simulink model "delta_dynamics"  (R2018a)
settings: Solver=VariableStepAuto  StartTime=0.0  StopTime=10.0  RelTol=1e-3
values from neighbouring files (symbols this model uses):
  Ig = [1 0 0; 0 1 0; 0 0 1]    [HapticsSetup.m]    (also in delta_massMatrix.m = u(1:3,:); delta_nonlinearTerm.m = u(1:3,:))
  M = m*eye(3)*Im    [HapticsSetup.m]    (also in Mmatrix.m = (J')^(-1)*Aq*(J^-1); delta_nonlinearTerm.m = u(4:6,:))
  q0 = [0;0;0]    [HapticsSetup.m]
  x0 = interx(p(:,1),p(:,2),p(:,3),Lb,Lb,Lb,0)    [HapticsSetup.m]
  xd0 = [0;0;0]    [HapticsSetup.m]
undefined symbols (not defined in the file or in its folder): delta_massMatrix, delta_nonlinearTerm, deltaJacobian, derivative_deltaInvJacobian
settings Model: Creator=klay  LastModifiedBy=augus
settings CodeAppCC: StateflowObjectComments=on

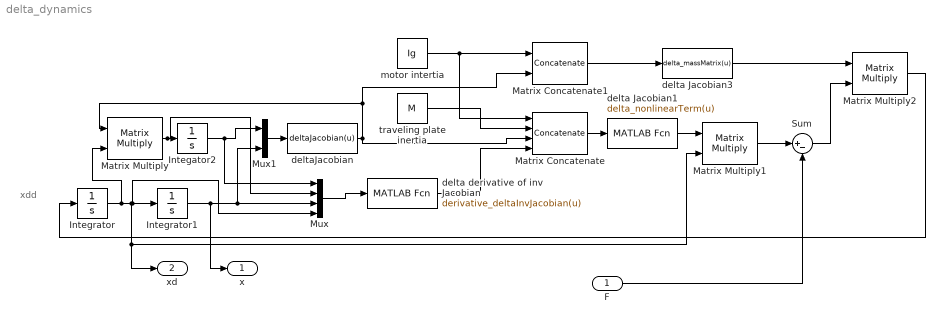
== system delta_dynamics ==
  note: xdd
  F : Inport  PortDimensions=3
  Integator2 : Integrator  InitialCondition=q0
  Integrator : Integrator  InitialCondition=xd0
  Integrator1 : Integrator  InitialCondition=x0
  Matrix Concatenate : Concatenate  NumInputs=4  Mode=Multidimensional array
  Matrix Concatenate1 : Concatenate  Mode=Multidimensional array
  Matrix Multiply : Product  Multiplication=Matrix(*)
  Matrix Multiply1 : Product  Multiplication=Matrix(*)
  Matrix Multiply2 : Product  Multiplication=Matrix(*)
  Mux : Mux
  Mux1 : Mux  Inputs=2
  Sum : Sum  Inputs=|+-
  delta Jacobian1 : MATLABFcn  MATLABFcn=delta_nonlinearTerm(u)  Output1D=off
  delta Jacobian3 : MATLABFcn  MATLABFcn=delta_massMatrix(u)  Output1D=off
  delta derivative of inv Jacobian : MATLABFcn  MATLABFcn=derivative_deltaInvJacobian(u)  Output1D=off
  deltaJacobian : MATLABFcn  MATLABFcn=deltaJacobian(u)  Output1D=off
  motor intertia : Constant  Value=Ig
  traveling plate inertia : Constant  Value=M
  x : Outport
  "xd " : Outport  Port=2
  wires:
  Matrix Multiply2/1 -> Integrator/1
  Matrix Multiply/1 -> Mux/2, Integator2/1
  Integrator/1 -> Matrix Multiply1/2, "xd "/1, Mux/4, Integrator1/1, Matrix Multiply/2
  deltaJacobian/1 -> Matrix Concatenate1/2, Matrix Multiply/1, Matrix Concatenate/3
  Matrix Concatenate/1 -> delta Jacobian1/1
  Mux/1 -> delta derivative of inv Jacobian/1
  delta derivative of inv Jacobian/1 -> Matrix Concatenate/4
  motor intertia/1 -> Matrix Concatenate1/1, Matrix Concatenate/1
  traveling plate inertia/1 -> Matrix Concatenate/2
  Matrix Concatenate1/1 -> delta Jacobian3/1
  delta Jacobian1/1 -> Matrix Multiply1/1
  Matrix Multiply1/1 -> Sum/1
  delta Jacobian3/1 -> Matrix Multiply2/1
  Sum/1 -> Matrix Multiply2/2
  Integrator1/1 -> Mux/3, Mux1/2, x/1
  Mux1/1 -> deltaJacobian/1
  Integator2/1 -> Mux/1, Mux1/1
  F/1 -> Sum/2
